simulink model "Zustandsregler"  (R2019b)
settings: Solver=FixedStepAuto  StartTime=0.0  StopTime=7  FixedStep=0.001  MaxStep=1e-3  RelTol=1e-3
values from neighbouring files (symbols this model uses):
  ausgangsVektor_cT = [0 , 1]    [init.m]    (also in matlab.mat = [1 1])
  durchgriffsVektor_d = [l , -lh/v]    [init.m]    (also in matlab.mat = [0.25 -0.0625])
  eingangsMatrix_B = [0 , 0 ; v, -1]    [init.m]    (also in matlab.mat = [0  0; 2  -1])
  regelMatrix_K = [b a ; b a]    [init.m]    (also in matlab.mat = [50  20; 50  20])
  systemMatrix_A = [0 , v ; 0 , 0]    [init.m]    (also in matlab.mat = [0  2; 0  0])
libraries: robotlib x6

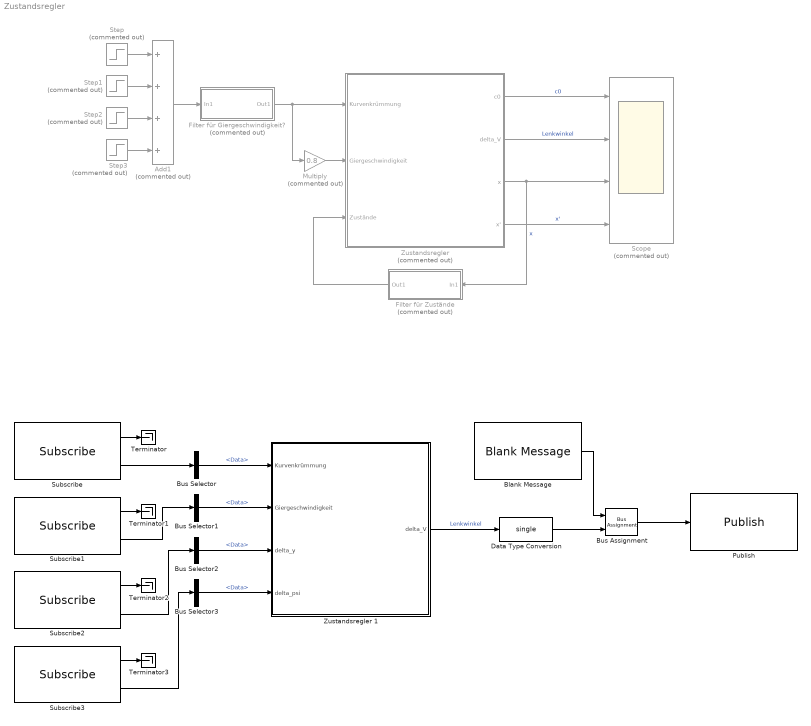
== system Zustandsregler ==
  Add1 : Sum  Commented=on  Inputs=++++
  Blank Message : robotlib/Blank Message  messageClass=Message  entityType=std_msgs/Float32  messageType=std_msgs/Float32  SampleTime=inf
  Bus Assignment : BusAssignment  AssignedSignals=Data
  Bus Selector{,1..3} (4 alike) : BusSelector  OutputSignals=Data
  Data Type Conversion : DataTypeConversion  OutDataTypeStr=single
  Filter für Giergeschwindigkeit? : Subsystem  Commented=on
  Filter für Zustände : Subsystem  Commented=on
  Multiply : Gain  Commented=on  Gain=0.8
  Publish : robotlib/Publish  topicSource=Specify your own  topic=/servolenkwinkel  messageType=std_msgs/Float32  messageQueueLength=1
  Scope : Scope  Commented=on  NumInputPorts=4
  Step : Step  Commented=on  SampleTime=0
  Step1 : Step  Commented=on  Time=1.75  After=-1  SampleTime=0
  Step2 : Step  Commented=on  Time=4  After=-1/1.5  SampleTime=0
  Step3 : Step  Commented=on  Time=6  After=1/1.5  SampleTime=0
  Subscribe : robotlib/Subscribe  topicSource=Specify your own  topic=/kurvenkruemmung  messageType=std_msgs/Float32  sampleTime=-1  messageQueueLength=1
  Subscribe1 : robotlib/Subscribe  topicSource=Specify your own  topic=/giergeschwindigkeit  messageType=std_msgs/Float32  sampleTime=-1  messageQueueLength=1
  Subscribe2 : robotlib/Subscribe  topicSource=Specify your own  topic=/spurmittenabstand  messageType=std_msgs/Float32  sampleTime=-1  messageQueueLength=1
  Subscribe3 : robotlib/Subscribe  topicSource=Specify your own  topic=/differenzwinkel  messageType=std_msgs/Float32  sampleTime=-1  messageQueueLength=1
  Terminator{,1..3} (4 alike) : Terminator
  "Zustandsregler " : Subsystem  Commented=on
  Zustandsregler 1 : Subsystem
  wires:
  Step/1 -> Add1/1
  Step1/1 -> Add1/2
  "Zustandsregler "/1(c0) -> Scope/1  "c0"
  "Zustandsregler "/2(delta_V) -> Scope/2  "Lenkwinkel"
  "Zustandsregler "/3(x) -> Filter für Zustände/1(In1), Scope/3  "x"
  "Zustandsregler "/4(x') -> Scope/4  "x'"
  Filter für Zustände/1(Out1) -> "Zustandsregler "/3(Zustände)
  Multiply/1 -> "Zustandsregler "/2("Giergeschwindigkeit ")
  Subscribe/2 -> Bus Selector/1
  Bus Selector/1 -> Zustandsregler 1/1("Kurvenkrümmung ")  "<Data>"
  Bus Selector1/1 -> Zustandsregler 1/2("Giergeschwindigkeit ")  "<Data>"
  Zustandsregler 1/1(delta_V) -> Data Type Conversion/1  "Lenkwinkel"
  Data Type Conversion/1 -> Bus Assignment/2
  Bus Assignment/1 -> Publish/1
  Blank Message/1 -> Bus Assignment/1
  Subscribe1/2 -> Bus Selector1/1
  Subscribe2/2 -> Bus Selector2/1
  Bus Selector2/1 -> Zustandsregler 1/3(delta_y)  "<Data>"
  Subscribe3/2 -> Bus Selector3/1
  Bus Selector3/1 -> Zustandsregler 1/4(delta_psi)  "<Data>"
  Step2/1 -> Add1/3
  Step3/1 -> Add1/4
  Add1/1 -> Filter für Giergeschwindigkeit?/1(In1)
  Filter für Giergeschwindigkeit?/1(Out1) -> Multiply/1, "Zustandsregler "/1("Kurvenkrümmung ")
  Subscribe/1 -> Terminator/1
  Subscribe3/1 -> Terminator3/1
  Subscribe2/1 -> Terminator2/1
  Subscribe1/1 -> Terminator1/1

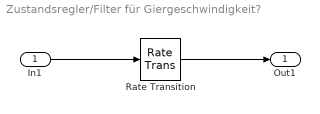
== system Zustandsregler/Filter für Giergeschwindigkeit? ==
  In1 : Inport
  Rate Transition : RateTransition  OutPortSampleTime=0.01
  Out1 : Outport
  wires:
  In1/1 -> Rate Transition/1
  Rate Transition/1 -> Out1/1

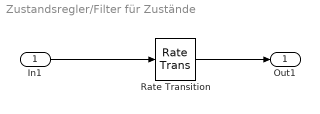
== system Zustandsregler/Filter für Zustände ==
  In1 : Inport
  Rate Transition : RateTransition  OutPortSampleTime=0.01
  Out1 : Outport
  wires:
  In1/1 -> Rate Transition/1
  Rate Transition/1 -> Out1/1

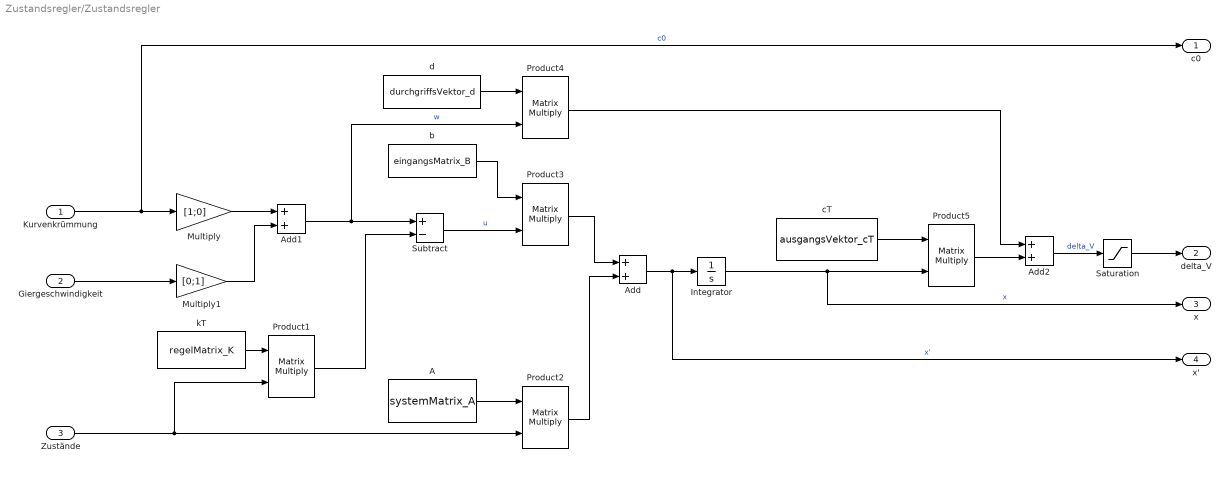
== system Zustandsregler/Zustandsregler  ==
  "Kurvenkrümmung " : Inport
  "Giergeschwindigkeit " : Inport  Port=2
  Zustände : Inport  Port=3
  A : Constant  Value=systemMatrix_A  VectorParams1D=off
  Add : Sum
  Add1 : Sum
  Add2 : Sum
  Integrator : Integrator
  Multiply : Gain  Gain=[1;0]
  Multiply1 : Gain  Gain=[0;1]
  Product{1..5} (5 alike) : Product  Multiplication=Matrix(*)
  Saturation : Saturate  UpperLimit=0.349  LowerLimit=-0.349
  Subtract : Sum  Inputs=+-
  b : Constant  Value=eingangsMatrix_B  VectorParams1D=off
  cT : Constant  Value=ausgangsVektor_cT  VectorParams1D=off
  d : Constant  Value=durchgriffsVektor_d  VectorParams1D=off
  kT : Constant  Value=regelMatrix_K  VectorParams1D=off
  c0 : Outport
  delta_V : Outport  Port=2
  x : Outport  Port=3
  x' : Outport  Port=4
  wires:
  Product1/1 -> Subtract/2
  cT/1 -> Product5/1
  Integrator/1 -> Product5/2, x/1  "x"
  Add/1 -> x'/1, Integrator/1  "x'"
  "Kurvenkrümmung "/1 -> Multiply/1, c0/1  "c0"
  A/1 -> Product2/1
  Product3/1 -> Add/1
  kT/1 -> Product1/1
  Add2/1 -> Saturation/1  "delta_V"
  b/1 -> Product3/1
  Subtract/1 -> Product3/2  "u"
  Multiply/1 -> Add1/1
  Add1/1 -> Product4/2, Subtract/1  "w"
  Multiply1/1 -> Add1/2
  Product2/1 -> Add/2
  "Giergeschwindigkeit "/1 -> Multiply1/1
  Zustände/1 -> Product1/2, Product2/2
  Saturation/1 -> delta_V/1
  d/1 -> Product4/1
  Product5/1 -> Add2/2
  Product4/1 -> Add2/1

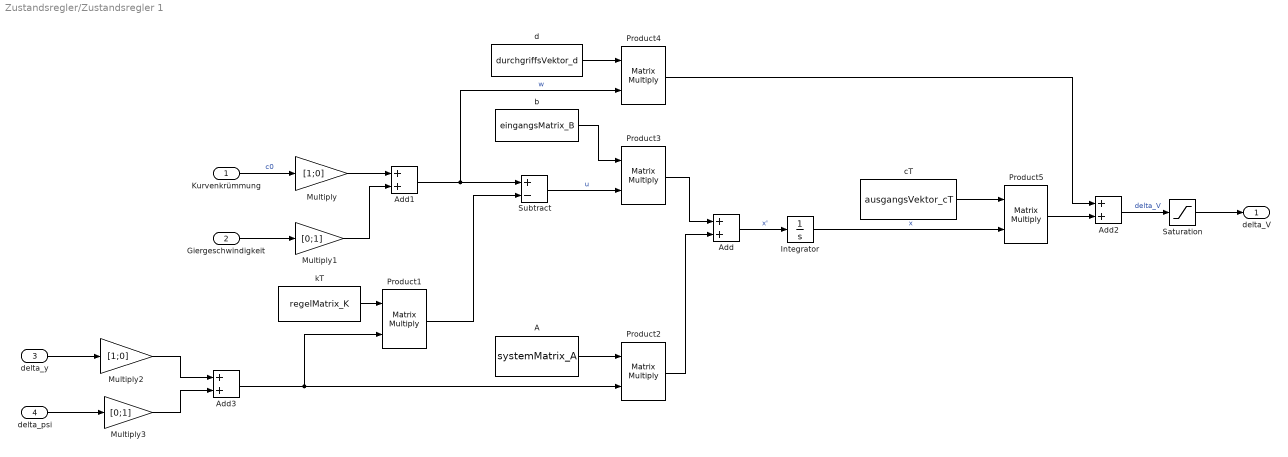
== system Zustandsregler/Zustandsregler 1 ==
  "Kurvenkrümmung " : Inport
  "Giergeschwindigkeit " : Inport  Port=2
  delta_y : Inport  Port=3
  delta_psi : Inport  Port=4
  A : Constant  Value=systemMatrix_A  VectorParams1D=off
  Add{,1..3} (4 alike) : Sum
  Integrator : Integrator
  Multiply : Gain  Gain=[1;0]
  Multiply1 : Gain  Gain=[0;1]
  Multiply2 : Gain  Gain=[1;0]
  Multiply3 : Gain  Gain=[0;1]
  Product{1..5} (5 alike) : Product  Multiplication=Matrix(*)
  Saturation : Saturate  UpperLimit=0.349  LowerLimit=-0.349
  Subtract : Sum  Inputs=+-
  b : Constant  Value=eingangsMatrix_B  VectorParams1D=off
  cT : Constant  Value=ausgangsVektor_cT  VectorParams1D=off
  d : Constant  Value=durchgriffsVektor_d  VectorParams1D=off
  kT : Constant  Value=regelMatrix_K  VectorParams1D=off
  delta_V : Outport
  wires:
  Product1/1 -> Subtract/2
  cT/1 -> Product5/1
  Integrator/1 -> Product5/2  "x"
  Add/1 -> Integrator/1  "x'"
  "Kurvenkrümmung "/1 -> Multiply/1  "c0"
  A/1 -> Product2/1
  Product3/1 -> Add/1
  kT/1 -> Product1/1
  Add2/1 -> Saturation/1  "delta_V"
  b/1 -> Product3/1
  Subtract/1 -> Product3/2  "u"
  Multiply/1 -> Add1/1
  Add1/1 -> Product4/2, Subtract/1  "w"
  Multiply1/1 -> Add1/2
  Product2/1 -> Add/2
  "Giergeschwindigkeit "/1 -> Multiply1/1
  delta_y/1 -> Multiply2/1
  Saturation/1 -> delta_V/1
  d/1 -> Product4/1
  Product5/1 -> Add2/2
  Product4/1 -> Add2/1
  Multiply2/1 -> Add3/1
  Multiply3/1 -> Add3/2
  Add3/1 -> Product1/2, Product2/2
  delta_psi/1 -> Multiply3/1
